simulink model "taskSplitTestbed"  (R2012b)
settings: Solver=FixedStepDiscrete  StartTime=0.0  StopTime=inf  RelTol=1e-3
settings Model: BufferReuse=off  ExplicitPartitioning=on  Creator=gilja  LastModifiedBy=NPTL
settings SolverCC: EnableConcurrentExecution=on  ConcurrentTasks=on
settings OptimizationCC: InlineParams=on  InlineInvariantSignals=on  OptimizeBlockIOStorage=off  BufferReuse=off  ExpressionFolding=off  LocalBlockOutputs=off
settings HardwareCC: ProdIntDivRoundTo=Zero  ProdEndianess=LittleEndian  ProdHWDeviceType=Generic->32-bit x86 compatible
settings ModelReferenceCC: ModelReferenceMinAlgLoopOccurrences=on
settings RTWCC: SystemTargetFile=xpctarget.tlc  TemplateMakefile=xpc_default_tmf  Description=xPC Target  ProcessScript=xpctarget_make_rtw_hook
settings CodeAppCC: MaxIdLength=62
settings xpcTargetCC: TargetFcnLib=ansi_tfl_table_tmw.mat  CodeReplacementLibrary=XPC_BLAS  ParMdlRefBuildCompliant=on  ConcurrentExecutionCompliant=on  CombineSignalStateStructs=off  GRTInterface=on  xPCTaskExecutionProfile=on  xPCRL32EventNumber=5000  RL32IRQSourceModifier=5  xPCIRQSourceBoard=Parallel_Port  xPCIOIRQSlot=0x378  xPCisDownloadable=off  xPCLoadParamSetFile=off  xPCConcurrentTasks=off  xPCEnableSFAnimation=off

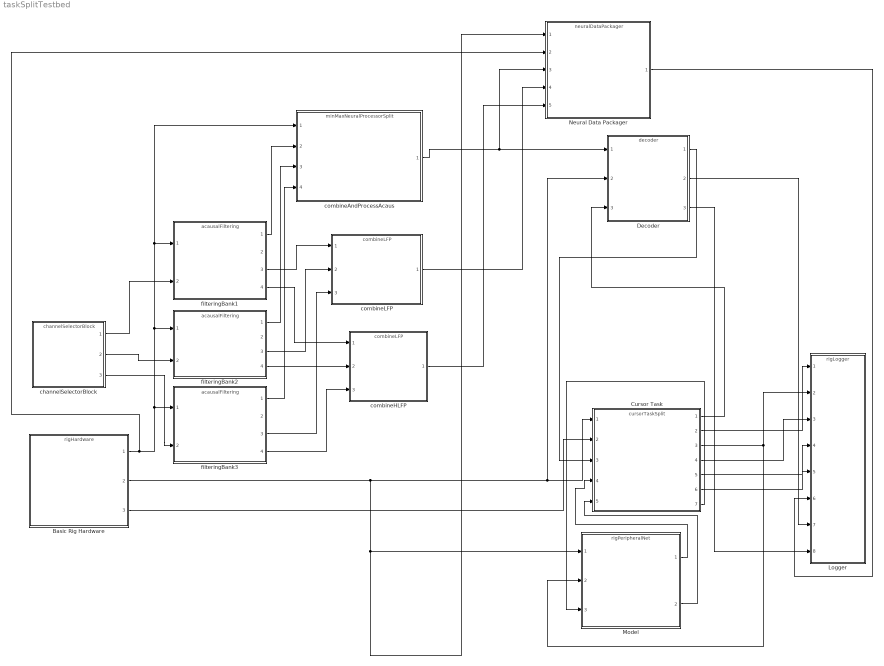
== system taskSplitTestbed ==
  Basic Rig Hardware : ModelReference  ModelNameDialog=rigHardware  SimulationMode=Normal  ModelReferenceVersion=1.64  CopyOfModelName=rigHardware  DefaultDataLogging=on
  Cursor Task : ModelReference  ModelNameDialog=cursorTaskSplit  SimulationMode=Normal  ModelReferenceVersion=1.207  CopyOfModelName=cursorTaskSplit  DefaultDataLogging=on
  Decoder : ModelReference  ModelNameDialog=decoder  SimulationMode=Normal  ModelReferenceVersion=1.141  CopyOfModelName=decoder  DefaultDataLogging=on
  Logger : ModelReference  ModelNameDialog=rigLogger  SimulationMode=Normal  ModelReferenceVersion=1.120  CopyOfModelName=rigLogger  DefaultDataLogging=on
  Model : ModelReference  ModelNameDialog=rigPeripheralNet  SimulationMode=Normal  ModelReferenceVersion=1.158  CopyOfModelName=rigPeripheralNet  DefaultDataLogging=on
  Neural Data Packager : ModelReference  ModelNameDialog=neuralDataPackager  SimulationMode=Normal  ModelReferenceVersion=1.147  CopyOfModelName=neuralDataPackager  DefaultDataLogging=on
  channelSelectorBlock : ModelReference  ModelNameDialog=channelSelectorBlock  SimulationMode=Normal  ModelReferenceVersion=1.35  CopyOfModelName=channelSelectorBlock  DefaultDataLogging=on
  combineAndProcessAcaus : ModelReference  ModelNameDialog=minMaxNeuralProcessorSplit  SimulationMode=Normal  ModelReferenceVersion=1.33  CopyOfModelName=minMaxNeuralProcessorSplit  DefaultDataLogging=on
  combineHLFP : ModelReference  ModelNameDialog=combineLFP  SimulationMode=Normal  ModelReferenceVersion=1.37  CopyOfModelName=combineLFP  DefaultDataLogging=on
  combineLFP : ModelReference  ModelNameDialog=combineLFP  SimulationMode=Normal  ModelReferenceVersion=1.37  CopyOfModelName=combineLFP  DefaultDataLogging=on
  filteringBank1 : ModelReference  ModelNameDialog=acausalFiltering  SimulationMode=Normal  ModelReferenceVersion=1.46  CopyOfModelName=acausalFiltering  DefaultDataLogging=on
  filteringBank2 : ModelReference  ModelNameDialog=acausalFiltering  SimulationMode=Normal  ModelReferenceVersion=1.46  CopyOfModelName=acausalFiltering  DefaultDataLogging=on
  filteringBank3 : ModelReference  ModelNameDialog=acausalFiltering  SimulationMode=Normal  ModelReferenceVersion=1.46  CopyOfModelName=acausalFiltering  DefaultDataLogging=on
  wires:
  Basic Rig Hardware/1 -> filteringBank2/1, combineAndProcessAcaus/1, filteringBank1/1, filteringBank3/1, Neural Data Packager/2
  filteringBank1/1 -> combineAndProcessAcaus/2
  channelSelectorBlock/1 -> filteringBank1/2
  channelSelectorBlock/2 -> filteringBank2/2
  filteringBank2/1 -> combineAndProcessAcaus/3
  channelSelectorBlock/3 -> filteringBank3/2
  filteringBank3/1 -> combineAndProcessAcaus/4
  filteringBank1/4 -> combineHLFP/1
  filteringBank2/4 -> combineHLFP/2
  filteringBank3/4 -> combineHLFP/3
  Basic Rig Hardware/2 -> Neural Data Packager/1, Model/1, Cursor Task/1, Decoder/2
  Basic Rig Hardware/3 -> Cursor Task/2
  combineAndProcessAcaus/1 -> Neural Data Packager/3, Decoder/1
  Decoder/1 -> Cursor Task/3
  Neural Data Packager/1 -> Logger/6
  Cursor Task/2 -> Logger/1
  Cursor Task/3 -> Logger/2, Model/2
  Cursor Task/4 -> Logger/3
  Cursor Task/5 -> Logger/4
  Cursor Task/6 -> Logger/5
  Cursor Task/7 -> Model/3
  Model/1 -> Cursor Task/4
  Model/2 -> Cursor Task/5
  Cursor Task/1 -> Decoder/3
  filteringBank1/3 -> combineLFP/1
  filteringBank2/3 -> combineLFP/2
  filteringBank3/3 -> combineLFP/3
  combineLFP/1 -> Neural Data Packager/4
  combineHLFP/1 -> Neural Data Packager/5
  Decoder/2 -> Logger/7
  Decoder/3 -> Logger/8
